simulink model "factory_cameratest"  (R2023a)
settings: Solver=FixedStepAuto  StartTime=0.0  StopTime=inf  RelTol=1e-3
undefined symbols (not defined in the file or in its folder): gray
libraries: mjLib x2
settings Model: Creator=vmano  LastModifiedBy=vmano
settings OptimizationCC: ReuseModelBlockBuffer=off
settings SFSimCC: SimTargetLang=C++

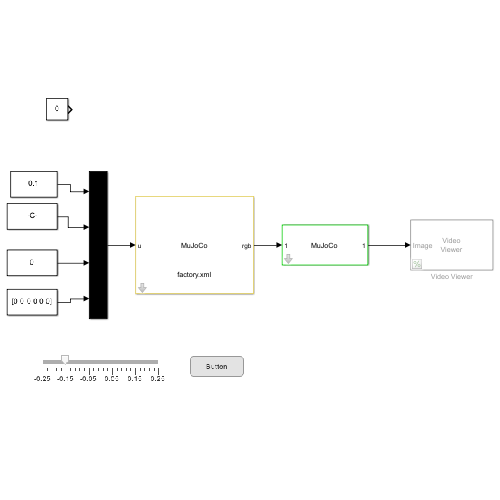
[thumbnail: Simulink's stored preview of the top-level diagram]
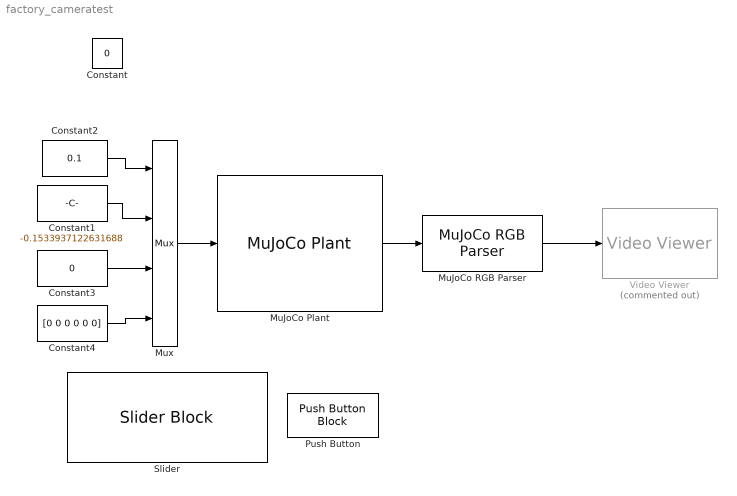
== system factory_cameratest ==
  Constant : Constant  Value=0
  Constant1 : Constant  Value=-0.1533937122631688
  Constant2 : Constant  Value=0.1
  Constant3 : Constant  Value=0
  Constant4 : Constant  Value=[0 0 0 0 0 0]
  MuJoCo Plant : mjLib/MuJoCo Plant  controlBus=[]  sensorBus=mj_bus_sensor_7979902499018342666  controlLength=[]  sensorLength=[]  rgbLength=[]  depthLength=[]  sampleTime=0.001  xmlFileRel=.\models\factory.xml  xmlFile=.\models\factory.xml  renderingType=Global  vsync=off  visualFPS=60  zoomLevel=1  znear=0.03  zfar=150  cameraSampleTime=0.040  rgbOutOption=on  depthOutOption=off  controlInterfaceType=Vector
      settings: SourceProductName=MuJoCo Simulator
  MuJoCo RGB Parser : mjLib/MuJoCo RGB Parser  inputBusType=mj_bus_rgb_6905886718754851708  selectedCamera=rgbcam  imageRows=480  imageCols=640  startingIndex=1  endingIndex=921600
      settings: SourceProductName=MuJoCo Simulator
  Mux : Mux
  Push Button : PushButtonBlock  OnValue=0.1  ButtonType=Latch  OffValue=0.010000
  Slider : SliderBlock  LabelPosition=Hide  ScaleMin=-0.25  ScaleMax=0.25
  Video Viewer : VideoViewer  Commented=on  colormapValue=gray(256)  FigPos=[2041 741.333333333333 418 304]
  wires:
  Mux/1 -> MuJoCo Plant/1
  Constant1/1 -> Mux/2
  Constant3/1 -> Mux/3
  Constant4/1 -> Mux/4
  MuJoCo Plant/1 -> MuJoCo RGB Parser/1
  MuJoCo RGB Parser/1 -> Video Viewer/1
  Constant2/1 -> Mux/1
